simulink model "xDamper"  (R2024b)
settings: configuration reference "STM32H7_Config" (kept outside this file)
undefined symbols (not defined in the file): xDamperGain, xDamperOffsetFL, xDamperOffsetFR, xDamperOffsetRL, xDamperOffsetRR
settings Model: DataDictionary=Master_Dictionary.sldd  EnableAccessToBaseWorkspace=off  Creator=torni  LastModifiedBy=William
settings ConfigSetRef: SourceName=STM32H7_Config

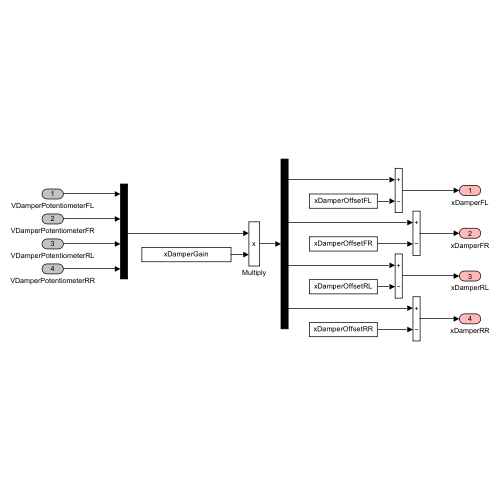
[thumbnail: Simulink's stored preview of the top-level diagram]
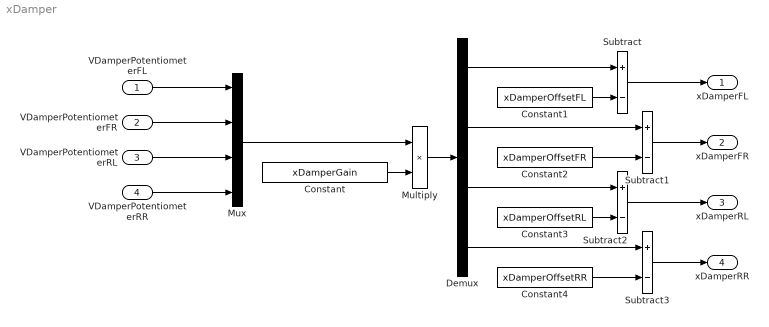
== system xDamper ==
  VDamperPotentiometerFL : Inport  OutDataTypeStr=double
  "VDamperPotentiometerFR " : Inport  Port=2  OutDataTypeStr=double
  VDamperPotentiometerRL : Inport  Port=3  OutDataTypeStr=double
  VDamperPotentiometerRR : Inport  Port=4  OutDataTypeStr=double
  Constant : Constant  Value=xDamperGain  SampleTime=-1
  Constant1 : Constant  Value=xDamperOffsetFL  SampleTime=-1
  Constant2 : Constant  Value=xDamperOffsetFR  SampleTime=-1
  Constant3 : Constant  Value=xDamperOffsetRL  SampleTime=-1
  Constant4 : Constant  Value=xDamperOffsetRR  SampleTime=-1
  Demux : Demux
  Multiply : Product
  Mux : Mux
  Subtract{,1..3} (4 alike) : Sum  Inputs=+-
  xDamperFL : Outport  OutDataTypeStr=double  VectorParamsAs1DForOutWhenUnconnected=off
  xDamperFR : Outport  Port=2  OutDataTypeStr=double  VectorParamsAs1DForOutWhenUnconnected=off
  xDamperRL : Outport  Port=3  OutDataTypeStr=double  VectorParamsAs1DForOutWhenUnconnected=off
  xDamperRR : Outport  Port=4  OutDataTypeStr=double  VectorParamsAs1DForOutWhenUnconnected=off
  wires:
  Demux/3 -> Subtract2/1
  Constant/1 -> Multiply/2
  VDamperPotentiometerRR/1 -> Mux/4
  VDamperPotentiometerRL/1 -> Mux/3
  VDamperPotentiometerFL/1 -> Mux/1
  Demux/2 -> Subtract1/1
  Constant4/1 -> Subtract3/2
  Demux/4 -> Subtract3/1
  Subtract2/1 -> xDamperRL/1
  Constant3/1 -> Subtract2/2
  Subtract3/1 -> xDamperRR/1
  Multiply/1 -> Demux/1
  Mux/1 -> Multiply/1
  Subtract1/1 -> xDamperFR/1
  Subtract/1 -> xDamperFL/1
  Demux/1 -> Subtract/1
  "VDamperPotentiometerFR "/1 -> Mux/2
  Constant2/1 -> Subtract1/2
  Constant1/1 -> Subtract/2
